simulink library "CommunicationSwitch"  (Simulink 7.4)
settings: Solver=ode45  StartTime=0.0  StopTime=10.0  RelTol=1e-3
settings Model: Creator=dread  LastModifiedBy=dread

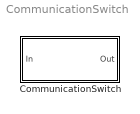
== system CommunicationSwitch ==
  CommunicationSwitch : Subsystem

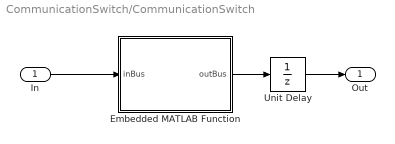
== system CommunicationSwitch/CommunicationSwitch ==
  In : Inport  UseBusObject=on  OutDataType=CommunicationBus
      settings: BusObject=RailCabBus
  Embedded MATLAB Function : Stateflow chart
  Unit Delay : UnitDelay  SampleTime=-1
  Out : Outport  OutDataType=CommunicationBus
  wires:
  Unit Delay/1 -> Out/1
  Embedded MATLAB Function/1(outBus) -> Unit Delay/1
  In/1 -> Embedded MATLAB Function/1(inBus)

== matlab function CommunicationSwitch/Embedded MATLAB Function ==
  data: inBus input Bus: RailCabBus; outBus output Bus: RailCabBus
function outBus = BusImpl(inBus)
%#eml
eml.extrinsic('fieldnames','disp','setfield','fprintf');

busSize = numel(inBus.rc1.from);
queueSize = 10*busSize; %length of queue
numShuttles = 0; %Define data type
numShuttles = numel(fieldnames(inBus)); %Shuttles connected to the bus
assert(numShuttles <= 20) %Defines an upper bound for number of shuttles. 
%Important for static memory allocation. 
lookupTableSize = 200;



NOT_ASSIGNED = -1;

%We need persistent queues
persistent queue;
persistent lookupTable;

%Initialize the queues
if isempty(queue)
    queue = repmat(emptyPacket(), numShuttles, queueSize);
end

if isempty(lookupTable)
    lookupTable = repmat(NOT_ASSIGNED, lookupTableSize,1);
end

%Clean outbus
outBus = inBus;
for i = 1:numShuttles
    outBus = setfield(outBus, createRailCabName(i), emptyBus(busSize));
end

%Retrieve packets
for i = 1:numShuttles
    %Get current bus
    currentBus = getBusFromIndex(inBus, busSize, i);
    for j = 1:busSize
        %Read packet
        packet = getPacketFromBus(currentBus, j);
        
        %Check if new packet
        if isValid(packet, numShuttles)
             %Save sender bus element to lookup table
            if lookupTable(packet.from) == NOT_ASSIGNED
                lookupTable(packet.from) = i;
            end
            
            %Save packet in queue
            target = lookupTable(packet.to);
            %Destination unkown. Send to all unassigned.
            if target == NOT_ASSIGNED
                for k = 1:numShuttles
                    if(lookupTable(k) == NOT_ASSIGNED)
                        queue(k,:) = enqueue(queue(k,:), packet); 
                    end
                end                
            %Destination known
            else 
                queue(target,:) = enqueue(queue(target,:), packet);
            end            
        end
    end

end

%Send packet from queue
for i = 1:numShuttles    
    currentBus = getBusFromIndex(outBus, busSize, i);
    for j = 1:busSize
        if ~isEmpty(queue(i,:))
            
            
            %Read last packet
            packet = front(queue(i,:));
            queue(i,:) = dequeue(queue(i,:)); 
            
%            if packet.msg ~= 255 %No ACK
%                fprintf('Sending on port %u[%u/%u]: %s\n', i, j, busSize, toString(packet));
%            end            
            
            %Save packet to bus
            currentBus = setPacketToBus(currentBus, j, packet);
            
        else
            break;
        end
    end 
    %Save bus
    outBus = setBusToIndex(outBus, i, currentBus);
end

%%%%%%%%%%%%%%%%%%%%%%%%%%%%%%%%%%%%%%%%%%%%%%%%%%%%%%%%%%%%%%%%%%%%%%%%%%%
%% BUS
%%%%%%%%%%%%%%%%%%%%%%%%%%%%%%%%%%%%%%%%%%%%%%%%%%%%%%%%%%%%%%%%%%%%%%%%%%%

function name = createRailCabName(index) %#eml
%Create name for the railcab used on the bus
eml.extrinsic('sprintf');
name = sprintf('rc%d', index);

function bus = getBusFromIndex(inBus, busSize, index) %eml
%Retrieve a PacketBus from the RailCaBbus
eml.extrinsic('getfield');
busName = createRailCabName(index);
bus = emptyBus(busSize);
bus = getfield(inBus, busName);

function rcBus = setBusToIndex(rcBus, index, packetBus) %eml
%Save a PacketBus to RailCabBus
eml.extrinsic('setfield');
busName = createRailCabName(index);
rcBus = setfield(rcBus, busName, packetBus);

function packet = getPacketFromBus(packetBus, index) %eml
%Retrieve a packet from the bus
packet = emptyPacket();
packet.from = packetBus.from(index);
packet.to = packetBus.to(index);
packet.msg = packetBus.msg(index);
packet.param = packetBus.param (index);
packet.pkgid = packetBus.pkgid(index);
packet.time = packetBus.time(index);

function packetBus = setPacketToBus(packetBus, index, packet) %eml
%Save a packet to the bus
packetBus.from(index) = packet.from;
packetBus.to(index) = packet.to;
packetBus.msg(index) = packet.msg;
packetBus.param (index) = packet.param;
packetBus.pkgid(index) = packet.pkgid;
packetBus.time(index) = packet.time;

function bus = emptyBus(size) %emp
%Create an empty bus
bus = struct('from', zeros(size,1,'uint8'),'to', zeros(size,1,'uint8'),'msg', zeros(size,1,'uint16'),'param', zeros(size,1,'double'),'pkgid', zeros(size,1,'uint32'), 'time', zeros(size,1,'double'));


%%%%%%%%%%%%%%%%%%%%%%%%%%%%%%%%%%%%%%%%%%%%%%%%%%%%%%%%%%%%%%%%%%%%%%%%%%%
%% PACKET
%%%%%%%%%%%%%%%%%%%%%%%%%%%%%%%%%%%%%%%%%%%%%%%%%%%%%%%%%%%%%%%%%%%%%%%%%%%
function packet = emptyPacket() %#eml
%Creates an empty packet
packet = struct('from', uint8(0),'to', uint8(0),'msg', uint16(0),'param', double(0.0),'pkgid', uint32(0), 'time', double(0));

function valid = isValid(packet, numShuttles) %#eml
%Checks wether the given packet is valid and transported by the bus
eml.extrinsic('getfield');
valid = false;
if packet.to > 0 && packet.to <= numShuttles 
    if packet.from > 0 && packet.from <= numShuttles
        valid = true;
    end
end

function packetString = toString(packet) %#eml
eml.extrinsic('sprintf');
packetString = sprintf('%3u: %u->%u :%3u (%.1f) @%.2f', packet.pkgid, packet.from, packet.to, packet.msg, packet.param, packet.time);

%%%%%%%%%%%%%%%%%%%%%%%%%%%%%%%%%%%%%%%%%%%%%%%%%%%%%%%%%%%%%%%%%%%%%%%%%%%
%% QUEUE
%%%%%%%%%%%%%%%%%%%%%%%%%%%%%%%%%%%%%%%%%%%%%%%%%%%%%%%%%%%%%%%%%%%%%%%%%%%

function queue = enqueue(queue, packet) %#eml
%Insert the packet at the end of the queue
eml.extrinsic('warning');
for i=1:length(queue)
    if queue(i).to == 0
        queue(i) = packet;
        return;
    end
end
%No empty entry found
warning('RailCab:Bus','Bus: buffer overflow for outgoing queue to %d', queue(1).to);

function queue = dequeue(queue) %#eml
%Removes the first packet of the queue
for i = 1:length(queue)-1
    queue(i) = queue(i+1);
    if queue(i).to == 0
        %end reached
        return;
    end
end
queue(length(queue)) = emptyPacket();

function packet = front(queue) %#eml
%Returns the first element from the queue
packet = queue(1);

function empty = isEmpty(queue) %#eml
%Checks whether the queue is empty or not
packet = queue(1);
if packet.to == 0
    empty = true;
else
    empty = false;
end
